simulink model "asbCubeSat"  (R2025b)
settings: Solver=VariableStepAuto  StartTime=0.0  StopTime=20000  FixedStep=CubeSatTimeStep  MaxStep=10  RelTol=1e-7  AbsTol=1e-7  EnableMultiTasking=on
undefined symbols (not defined in the file): CubeSatTimeStep
libraries: simulink x12, aerolibutil x9, simulink_extras x3, asbCubeSatEnvironmentLib x1, SignalEditorBlockLib x1, sharedutil x1, asbCubeSatActuatorsLib x1, asbCubeSatSensorsLib x1, aerolibattitudesys x1, aerolibtransform2 x1
(part 2 of 2)

== matlab function asbCubeSat/Vehicle Model/MATLAB Function ==
  settings: updateMethod=DISCRETE  sampleTime=0.1
  data: estimate_err_body output; deg_error output; w_est output; q_est output; q_b2eci input; w_eci2b input; bias output; reference_mag input; m output
function [estimate_err_body, deg_error, w_est, q_est, bias, m] = fcn(q_b2eci, w_eci2b, reference_mag)
    % --- Constants & Sensor Specs ---
    dt = 0.1;

    % Fix #9: timestep_per_mode now matches switch_every in
    % ukf_python_replica.m ( = int(60*10/dt) = 6000 ). Was 10000, which
    % did not correspond to anything in the reference implementation.
    timestep_per_mode = int32(60 * 45 / dt);

    % Truth gyro error model -- matches true_gyro_bias in
    % ukf_python_replica.m (fix #2: previously the bias truth was zero, so
    % the filter had nothing real to estimate). Scale factor has been
    % pulled out of both the truth model and the filter state -- see the
    % removal note near the state-vector definition below.
    true_gyro_bias    = [0.002, -0.001, 0.0015];

    % REVERTED (per empirical observation): the Python-matched sigmas
    % (gyro_noise=0.0005, measurement_noise=0.05) converged worse in
    % practice than these original values, so noise tuning is reverted to
    % match the original Simulink file exactly. This intentionally
    % diverges from the current sigma_gyro/sigma_magnetometer in
    % ukf_python_replica.m -- if the Python file gets re-synced later,
    % re-check this against it rather than assuming they still match.
    gyro_noise        = 0.001;   % rad/s
    measurement_noise = 0.01;    % uT

    % Second reference vector for the 2-vector ("Sun+Mag") mode. Fixed
    % placeholder ECI unit vector for now (matches ref_vec_2 in
    % ukf_python_replica.m) -- NOT read from an actual sun sensor/ephemeris
    % yet. Swap this out for a real ECI sun vector once one is wired into
    % this block as an input.
    ref_vec_2_eci = [1, 0, 0];
    sigma_unit_vector = 0.01;   % second-vector sensor noise std, matches ukf_python_replica.m

    reference_mag = reshape(reference_mag/1000, [1,3]); % nT -> uT

    % --- Persistent State Memory ---
    persistent timestep mode error_state error_cov attitude_estimate;
    persistent true_body_to_ref_prev;

    if isempty(timestep)
        timestep = 0;
    end
    if isempty(mode)
        mode = 0; % 0: Sun+Mag (Full Observability, 2-vector), 1: Mag Only (Eclipse, 1-vector)
    end

    % 6-state error vector: [Attitude (3), Bias (3)]
    % Scale factor removed from the filter state -- it was estimating an
    % unobserved/unneeded 9th-order term for this use case. n = length(x)
    % is used everywhere downstream (calculate_lambda, get_sigma_points,
    % get_weights, iterate) rather than a hardcoded 9, so shrinking this to
    % 6 automatically resizes lambda, alpha/beta-derived weights, and the
    % 2n+1 = 13 sigma points -- no other change needed in those functions.
    if isempty(error_state)
        error_state = zeros([1,6]);
    end

    if isempty(error_cov)
        error_cov = eye(6, 6) * 0.01;
        error_cov(4:6,4:6) = eye(3)*2.5e-5;
    end

    % --- True Environment Simulation ---
    % Fix #10: q_eci2b arrives in this codebase's own "body->ref" sense
    % (i.e. the sense that apply_rotation's sandwich convention expects),
    % not "ref->body" as originally assumed here. Confirmed empirically
    % against a full external trajectory log: reconstructing angular
    % velocity from consecutive q_eci2b samples via
    % true_body_to_ref_prev^-1 * true_body_to_ref matched the logged
    % w_eci2b on 100% of the 60 dynamically-active steps (out of 8859
    % total consecutive-pair steps checked), with every alternative
    % assignment/ordering getting the sign backwards on all of them.
    % true_body_to_ref is therefore taken directly from the input, and
    % true_ref_to_body is derived from it by inversion (not the reverse).
    true_body_to_ref = Quaternion(real(q_b2eci)).quaternion_normalize();
    true_ref_to_body = true_body_to_ref.quaternion_inverse();

    if isempty(true_body_to_ref_prev)
        true_body_to_ref_prev = true_body_to_ref;  % first call: no history yet -> zero rate
    end
    % delta_q = true_body_to_ref_prev.quaternion_inverse().quaternion_multiply(true_body_to_ref);
    % true_angular_velocity = delta_q.quaternion2rotation_vec() / dt;
    % output = (reshape(true_angular_velocity, [1 3]) - reshape(w_eci2b, [1 3]));
    
    % Use the given w_eci2b from Simulink
    true_angular_velocity = w_eci2b;

    if isempty(attitude_estimate)
        attitude_estimate = true_body_to_ref;
    end

    % --- Rate Cadence ---
    % This block runs at 10 Hz (dt = 0.1s). Vector measurements are only
    % available/applied at 0.1 Hz -- once every (1/0.1)/dt = 100 calls --
    % matching the propagate-every-call/update-every-100th-call scheme in
    % ukf_python_replica.m (update_every = int(10/dt) = 100).
    measurement_rate_hz = 0.1;
    steps_per_measurement = round((1 / measurement_rate_hz) / dt);  % = 100
    do_update = (mod(timestep, steps_per_measurement) == 0);

    % Sensor readings
    % Fix #2: truth gyro measurement now matches ukf_python_replica.m --
    % true rate + true bias + (true scale factor .* true rate) + noise,
    % instead of just true rate + noise with a zero bias and no scale factor.
    gyro_measurement_noise = normrnd(0, gyro_noise, [1,3]);
    simulated_gyro_measurement = true_angular_velocity + true_gyro_bias + gyro_measurement_noise;

    % --- Reference Vector(s) & R sizing -- mode-dependent ---
    % mode == 0: "Sun+Mag" / 2-vector (full observability) -- stack the
    %            magnetometer with the second reference vector.
    % mode == 1: "Mag Only" / 1-vector (eclipse) -- magnetometer alone.
    % This mirrors ukf_python_replica.m's vector_input toggle (1 <-> 2),
    % which also swaps every switch_every steps via the same mode/timestep
    % machinery already in this file (see timestep_per_mode below).
    use_two_vector = (mode == 0);

    if use_two_vector
        ref_readings = [reference_mag / norm(reference_mag); ...
                         ref_vec_2_eci / norm(ref_vec_2_eci)];
        R = blkdiag(eye(3) * 2e-5, eye(3) * sigma_unit_vector^2);
    else
        ref_readings = reference_mag / norm(reference_mag);
        R = eye(3) * 2e-5;
    end

    if do_update
        % Only sample fresh vector readings when one is actually available
        % at the 0.1 Hz measurement rate.
        body_mag = true_ref_to_body.apply_rotation(reference_mag) + normrnd([0,0,0], measurement_noise);
        mag_unit = body_mag / norm(body_mag);

        if use_two_vector
            body_vec2 = true_ref_to_body.apply_rotation(ref_vec_2_eci) + normrnd([0,0,0], sigma_unit_vector);
            vec2_unit = body_vec2 / norm(body_vec2);
            body_msmts = [mag_unit, vec2_unit];
        else
            body_msmts = mag_unit;
        end
    else
        % unused: iterate() skips the correction step when do_update is
        % false. Sized to match ref_readings/R for the current mode so the
        % call below always has consistent argument shapes.
        body_msmts = zeros(1, size(ref_readings, 1) * 3);
    end

    % --- Q Matrix (Process Noise Tuning) ---
    % REVERTED (per empirical observation): back to the original fixed
    % constants rather than the gyro_noise-derived value, since the
    % original tuning converged better in practice. No longer claims to
    % match global_Q in ukf_python_replica.m -- see note above.
    Q = zeros(6,6);
    Q(1:3,1:3) = eye(3) * 4e-6;    % Attitude noise
    Q(4:6,4:6) = eye(3) * 1e-10;   % Bias random walk

    % --- UKF Iteration ---
    [error_state, attitude_estimate, error_cov] = iterate(error_state, attitude_estimate, error_cov, ...
        ref_readings, body_msmts, simulated_gyro_measurement, Q, R, dt, do_update);

    % --- TRUE STATE MEMORY FIX ---
    % Reset ONLY the attitude error (1:3) to zero after it's injected into the nominal quaternion.
    % Bias (4:6) persists naturally through the persistent variable.
    error_state(1:3) = [0 0 0];

    % --- Outputs & Loop Maintenance ---
    estimate_err_body = rad2deg(Quaternion.quat_diff(true_ref_to_body, attitude_estimate.quaternion_inverse()));
    q_est = attitude_estimate.to_array();
    deg_error = norm(estimate_err_body);
    bias = reshape(error_state(4:6), [1 3]); % Extract bias for logging
    
    w_est = simulated_gyro_measurement - bias;

    true_body_to_ref_prev = true_body_to_ref;
    timestep = timestep + 1;
    m = mode;

    if(mod(timestep, timestep_per_mode) == 0)
        if(mode == 1)
            mode = 0;
        else
            mode = 1;
        end
    end
end

% =========================================================================
% UKF HELPER FUNCTIONS -- exact translations of ukf_python_replica.m
% =========================================================================

function [new_error_state, new_guess, new_cov] = iterate(current_error_state, current_guess, current_cov,...
    ref_readings, body_msmts, gyro, Q, R, dt, do_update)

    n = length(current_error_state); % 6-state filter (attitude + bias)
    alpha = 0.1;
    beta = 2;

    % Fix #1: guard incoming covariance before building sigma points,
    % matching ensure_positive_definite(P) call at the top of
    % ukf_python_replica.m's iterate().
    current_cov = ensure_positive_definite(current_cov);

    lam = calculate_lambda(alpha, current_error_state);
    sigmas = get_sigma_points(lam, current_error_state, current_cov);
    quat_sigmas = error_sigmas_to_quat_sigmas(sigmas, current_guess);
    propagated_quat_sigmas = propagate_quat_sigmas(quat_sigmas, gyro, dt);   % always propagate (10 Hz)

    [covariance_weights, mean_weights] = get_weights(lam, current_error_state, alpha, beta);

    num_sigmas = size(propagated_quat_sigmas, 1);
    quaternions_of_propagated_sigmas = cell(num_sigmas, 1);
    for i = 1:num_sigmas
        quaternions_of_propagated_sigmas{i} = Quaternion(propagated_quat_sigmas(i, 1:4));
    end

    [average_quaternion, propagated_error_vectors] = gradient_descent( ...
        quaternions_of_propagated_sigmas, current_guess, mean_weights);

    propagated_errors = [propagated_error_vectors, propagated_quat_sigmas(:, 5:7)];

    mean_error = zeros(1, n);
    for col = 1:n
        var_mean = 0;
        for row = 1:num_sigmas
            var_mean = var_mean + propagated_errors(row, col) * mean_weights(row);
        end
        mean_error(col) = var_mean;
    end

    P_hat = zeros(n, n);
    for i = 1:num_sigmas
        err = propagated_errors(i, :) - mean_error;
        P_hat = P_hat + covariance_weights(i) * (err' * err);
    end
    P_hat = P_hat + Q;   % process noise always accrues, every propagate step

    if do_update
        % --- MEASUREMENT CORRECTION (only on 0.1 Hz update steps) ---
        measurements = get_measurements(propagated_quat_sigmas, ref_readings);

        msmt_size = size(measurements, 2);
        mean_measurement = zeros(1, msmt_size);
        for col = 1:msmt_size
            var_mean = 0;
            for row = 1:num_sigmas
                var_mean = var_mean + measurements(row, col) * mean_weights(row);
            end
            mean_measurement(col) = var_mean;
        end

        P_xz = zeros(n, msmt_size);
        for i = 1:num_sigmas
            err = propagated_errors(i, :) - mean_error;
            msmt_err = measurements(i, :) - mean_measurement;
            P_xz = P_xz + covariance_weights(i) * (err' * msmt_err);
        end

        P_zz = zeros(msmt_size, msmt_size);
        for i = 1:num_sigmas
            msmt_err = measurements(i, :) - mean_measurement;
            P_zz = P_zz + covariance_weights(i) * (msmt_err' * msmt_err);
        end

        P_vv = P_zz + R;
        k = P_xz * inv(P_vv);
        x_hat = mean_error + (k * (body_msmts - mean_measurement)')';

        % Matches ukf_python_replica.m exactly: P_hat - k @ P_vv @ k.T
        P = P_hat - k * P_vv * k';
    else
        % --- PREDICT-ONLY (propagate mean/covariance, no correction) ---
        x_hat = mean_error;
        P = P_hat;
    end

    % Fix #1: guard outgoing covariance after the update, matching
    % ensure_positive_definite(P) call at the end of
    % ukf_python_replica.m's iterate().
    P = ensure_positive_definite(P);

    x_hat_rot = Quaternion.rotation_vec2quaternion(x_hat(1:3));
    new_error_state = x_hat;
    new_guess = x_hat_rot.quaternion_multiply(average_quaternion);
    new_cov = P;
end

function P = ensure_positive_definite(P, epsilon)
    % Exact port of ensure_positive_definite() from ukf_python_replica.m
    if nargin < 2
        epsilon = 1e-9;
    end
    P = (P + P') / 2;
    % real() forces this to stay a real-typed array for codegen: eig() on a
    % generic square matrix is typed as potentially complex by MATLAB
    % Coder/Simulink even though P is symmetric here, which otherwise
    % causes "Cannot assign a complex value into a non-complex location."
    eigvals = real(eig(P));
    if min(eigvals) < epsilon
        P = P + eye(size(P,1)) * (epsilon - min(eigvals) + epsilon);
    end
end

function lam = calculate_lambda(alpha, x)
    n = length(x);
    kappa = 0;
    lam = alpha^2 * (n + kappa) - n;
end

function sigmas = get_sigma_points(lam, x, P)
    n = length(x);
    P = (P + P') / 2;
    P = P + eye(n) * 1e-10;
    U = chol((lam + n) * P);   % upper-triangular, U'*U = (lam+n)*P

    sigmas = zeros(2*n + 1, n);
    sigmas(1, :) = x;
    for k = 1:n
        sigmas(k + 1, :) = x + U(k, :);
    end
    for k = (n+1):(2*n)
        idx = k - n;
        sigmas(k + 1, :) = x - U(idx, :);
    end
end

function [covariance_weights, mean_weights] = get_weights(lam, x, alpha, beta)
    n = length(x);
    c = 0.5 / (n + lam);
    covariance_weights = ones(1, 2*n + 1) * c;
    mean_weights = ones(1, 2*n + 1) * c;
    covariance_weights(1) = lam / (n + lam) + (1 - alpha^2 + beta);
    mean_weights(1) = lam / (n + lam);
end

function quat_sigmas = error_sigmas_to_quat_sigmas(error_sigmas, rotation)
    n = size(error_sigmas, 1);
    quat_sigmas = zeros(n, 7);
    for i = 1:n
        quat_rot = Quaternion.rotation_vec2quaternion(error_sigmas(i, 1:3));
        new_quat_rot = quat_rot.quaternion_multiply(rotation);
        new_quat_rot = new_quat_rot.quaternion_normalize();
        quat_sigmas(i, :) = [new_quat_rot.to_array(), error_sigmas(i, 4:6)];
    end
end

function new_sigmas = propagate_quat_sigmas(quat_sigmas, gyro_measurement, dt)
    n = size(quat_sigmas, 1);
    new_sigmas = zeros(n, 7);
    for i = 1:n
        quaternion = quat_sigmas(i, 1:4);
        bias = quat_sigmas(i, 5:7);

        w = gyro_measurement - bias;

        new_quaternion = Quaternion(quaternion).quaternion_multiply( ...
    Quaternion.rotation_vec2quaternion(w * dt));
        new_quaternion = new_quaternion.quaternion_normalize();

        new_sigmas(i, :) = [new_quaternion.to_array(), quat_sigmas(i, 5:7)];
    end
end

function measurements = get_measurements(quat_sigmas, ref_vecs)
    % ref_vecs: k x 3 matrix, one ECI reference unit vector per row (k=1
    % for mag-only mode, k=2 for the 2-vector "Sun+Mag" mode). Produces a
    % 3*k-wide row per sigma point, concatenating each vector's rotated
    % body-frame prediction in the same order as ref_vecs' rows -- mirrors
    % ukf_python_replica.m's get_measurements() when ref_vecs is a list.
    n = size(quat_sigmas, 1);
    k = size(ref_vecs, 1);
    measurements = zeros(n, 3*k);
    for i = 1:n
        quat = Quaternion(quat_sigmas(i, 1:4));
        ECI_to_body = quat.quaternion_inverse();
        for j = 1:k
            measurements(i, (3*j-2):(3*j)) = ECI_to_body.apply_rotation(ref_vecs(j, :));
        end
    end
end

function error_vectors = get_error_vectors(Y, x)
    n = length(Y);
    error_vectors = zeros(n, 3);
    x_inv = x.quaternion_inverse();
    for i = 1:n
        error_quaternion = Y{i}.quaternion_multiply(x_inv);
        error_vectors(i, :) = error_quaternion.quaternion2rotation_vec();
    end
end

function [x, error_vectors] = gradient_descent(Y, x, weights)
    n_pts = length(Y);
    if nargin < 3 || isempty(weights)
        weights = ones(1, n_pts) / n_pts;
    end
    w = weights(:) / sum(weights);   % keep the negative centre weight
    for iter = 1:100
        error_vectors = get_error_vectors(Y, x);
        ave = sum(error_vectors .* w, 1);
        if norm(ave) < 1e-9
            break;
        end
        x = Quaternion.rotation_vec2quaternion(ave).quaternion_multiply(x);
    end
end

== matlab function asbCubeSat/Vehicle Model/Magnosphere Model ==
  data: r_ECI input size=[3,1]; B_ECI output size=[3,1]; JD input
% NOTE: I do not truly understand this algorithm, but it seems to work and
% gives accurate results with the example cases

function B_ECI = wmmECI_embedded(r_ECI, JD)
% wmmECI_embedded  Earth's magnetic field (ECI) using embedded WMM2025 coefficients
%
% Inputs:
%   r_ECI - [3x1] ECI position (m)
%   JD    - Julian Date
%
% Output:
%   B_ECI - [3x1] magnetic field in nT (ECI)
%
% Reference: NOAA WMM2025 (epoch 2025.0)
% --- Convert Julian date to decimal year (keep for potential use) ---
year = 2000 + (JD - 2451545.0) / 365.25;

% --- WMM2025 embedded Gauss coefficients (nT) ---
[g,h,gdot,hdot] = loadWMM2025();

% --- Extrapolate coefficients to given year (epoch 2025.0) ---
epoch = 2025.0;
decimalYear = jd2year(JD);
g = g + (decimalYear - epoch) .* gdot;
h = h + (decimalYear - epoch) .* hdot;

% --- Compute magnetic field in ECI ---
B_ECI = computeWMMfieldFromCoeffs_manual(r_ECI, g, h, JD);

end

%% ---------------------- coefficient loader (unchanged data) ----------------------
function [g, h, gdot, hdot] = loadWMM2025()
% loadWMM2025  Embedded WMM2025 coefficients
% Output arrays: g(n+1,m+1), h(n+1,m+1), gdot(n+1,m+1), hdot(n+1,m+1)
% Units: nT and nT/yr

data = [...
 1  0  -29351.8    0.0      12.0      0.0
 1  1  -1410.8   4545.4      9.7    -21.5
 2  0  -2556.6    0.0     -11.6      0.0
 2  1   2951.1  -3133.6     -5.2    -27.7
 2  2   1649.3   -815.1     -8.0    -12.1
 3  0   1361.0    0.0       -1.3      0.0
 3  1  -2404.1    -56.6     -4.2      4.0
 3  2   1243.8    237.5      0.4     -0.3
 3  3    453.6   -549.5    -15.6     -4.1
 4  0    895.0     0.0      -1.6      0.0
 4  1    799.5    278.6     -2.4     -1.1
 4  2     55.7   -133.9     -6.0      4.1
 4  3   -281.1    212.0      5.6      1.6
 4  4     12.1   -375.6     -7.0     -4.4
 5  0   -233.2     0.0       0.6      0.0
 5  1    368.9     45.4      1.4     -0.5
 5  2    187.2    220.2      0.0      2.2
 5  3   -138.7   -122.9      0.6      0.4
 5  4   -142.0     43.0      2.2      1.7
 5  5     20.9    106.1      0.9      1.9
 6  0     64.4     0.0      -0.2      0.0
 6  1     63.8    -18.4     -0.4      0.3
 6  2     76.9     16.8      0.9     -1.6
 6  3   -115.7     48.8      1.2     -0.4
 6  4    -40.9    -59.8     -0.9      0.9
 6  5     14.9     10.9      0.3      0.7
 6  6    -60.7     72.7      0.9      0.9
 7  0     79.5     0.0      -0.0      0.0
 7  1    -77.0    -48.9     -0.1      0.6
 7  2     -8.8    -14.4     -0.1      0.5
 7  3     59.3     -1.0      0.5     -0.8
 7  4     15.8     23.4     -0.1      0.0
 7  5      2.5     -7.4     -0.8     -1.0
 7  6    -11.1    -25.1     -0.8      0.6
 7  7     14.2     -2.3      0.8     -0.2
 8  0     23.2     0.0      -0.1      0.0
 8  1     10.8     7.1       0.2     -0.2
 8  2    -17.5    -12.6      0.0      0.5
 8  3      2.0     11.4      0.5     -0.4
 8  4    -21.7     -9.7     -0.1      0.4
 8  5     16.9     12.7      0.3     -0.5
 8  6     15.0      0.7      0.2     -0.6
 8  7    -16.8     -5.2     -0.0      0.3
 8  8      0.9      3.9      0.2      0.2
 9  0      4.6      0.0     -0.0      0.0
 9  1      7.8    -24.8     -0.1     -0.3
 9  2      3.0     12.2      0.1      0.3
 9  3     -0.2      8.3      0.3     -0.3
 9  4     -2.5     -3.3     -0.3      0.3
 9  5    -13.1     -5.2      0.0      0.2
 9  6      2.4      7.2      0.3     -0.1
 9  7      8.6     -0.6     -0.1     -0.2
 9  8     -8.7      0.8      0.1      0.4
 9  9    -12.9     10.0     -0.1      0.1
 10 0     -1.3      0.0      0.1      0.0
 10 1     -6.4      3.3      0.0      0.0
 10 2      0.2      0.0      0.1     -0.0
 10 3      2.0      2.4      0.1     -0.2
 10 4     -1.0      5.3     -0.0      0.1
 10 5     -0.6     -9.1     -0.3     -0.1
 10 6     -0.9      0.4      0.0      0.1
 10 7      1.5     -4.2     -0.1      0.0
 10 8      0.9     -3.8     -0.1     -0.1
 10 9     -2.7      0.9     -0.0      0.2
 10 10    -3.9     -9.1     -0.0     -0.0
 11 0      2.9      0.0      0.0      0.0
 11 1     -1.5      0.0     -0.0     -0.0
 11 2     -2.5      2.9      0.0      0.1
 11 3      2.4     -0.6      0.0     -0.0
 11 4     -0.6      0.2      0.0      0.1
 11 5     -0.1      0.5     -0.1     -0.0
 11 6     -0.6     -0.3      0.0     -0.0
 11 7     -0.1     -1.2     -0.0      0.1
 11 8      1.1     -1.7     -0.1     -0.0
 11 9     -1.0     -2.9     -0.1      0.0
 11 10    -0.2     -1.8     -0.1      0.0
 11 11     2.6     -2.3     -0.1      0.0
 12 0     -2.0      0.0      0.0      0.0
 12 1     -0.2     -1.3      0.0     -0.0
 12 2      0.3      0.7     -0.0      0.0
 12 3      1.2      1.0     -0.0     -0.1
 12 4     -1.3     -1.4     -0.0      0.1
 12 5      0.6     -0.0     -0.0      -0.0
 12 6      0.6      0.6      0.1     -0.0
 12 7      0.5     -0.1     -0.0     -0.0
 12 8     -0.1      0.8      0.0      0.0
 12 9     -0.4      0.1      0.0     -0.0
 12 10    -0.2     -1.0     -0.1     -0.0
 12 11    -1.3      0.1     -0.0      0.0
 12 12    -0.7      0.2     -0.1     -0.1 ];

maxN = max(data(:,1));
g = zeros(maxN+1);
h = zeros(maxN+1);
gdot = zeros(maxN+1);
hdot = zeros(maxN+1);

for i = 1:size(data,1)
    n = data(i,1);
    m = data(i,2);
    g(n+1,m+1) = data(i,3);
    h(n+1,m+1) = data(i,4);
    gdot(n+1,m+1) = data(i,5);
    hdot(n+1,m+1) = data(i,6);
end
end

%% ---------------------- core compute routine ----------------------
function B_ECI = computeWMMfieldFromCoeffs_manual(r_ECI, g, h, jd)
    % Convert ECI -> ECEF
    theta = gmst_from_jd(jd);
    Rz = [ cos(theta)  sin(theta) 0;
          -sin(theta)  cos(theta) 0;
             0           0        1];

    r_ecef = Rz * r_ECI(:);

  

    % ECEF -> geodetic (WGS84)
    [lat, lon, alt] = ecef2geodetic(r_ecef);
    
    % Synthesize magnetic field in NED (nT)
    [B_north, B_east, B_down] = synthesizeMagField_manual(lat, lon, alt, g, h);

    % NED -> ECEF (NED vector to ECEF vector)
    R_ned2ecef = [ -sin(lat)*cos(lon), -sin(lat)*sin(lon),  cos(lat);
                   -sin(lon),            cos(lon),           0;
                   -cos(lat)*cos(lon),  -cos(lat)*sin(lon), -sin(lat)];
    B_ecef = R_ned2ecef * [B_north; B_east; B_down];
    
    B_ECI = Rz' * B_ecef;    % still in nT
end
%% ---------------------- Decyear -------------------------------------
function dyear = decyear_cg(year, month, day, hour, minute, second)
%DECYEAR_CG Codegen-compatible decimal year calculation
%   dyear = decyear_cg(year, month, day, hour, minute, second)
%   Equivalent to MATLAB's decyear(), but usable in code generation.

    if nargin < 6, second = 0; end
    if nargin < 5, minute = 0; end
    if nargin < 4, hour   = 0; end

    % Days in each month (non-leap year baseline)
    daysInMonth = [31 28 31 30 31 30 31 31 30 31 30 31];

    % Leap year check (Gregorian rule)
    isLeap = (mod(year,4)==0 && mod(year,100)~=0) || (mod(year,400)==0);
    if isLeap
        daysInMonth(2) = 29;
    end

    % Total days in the year
    if isLeap
        totalDays = 366;
    else
        totalDays = 365;
    end

    % Day of year (integer part)
    dayOfYear = sum(daysInMonth(1:month-1)) + day;

    % Fractional day from time-of-day
    fracDay = (hour + minute/60 + second/3600) / 24;

    % Decimal year
    dyear = year + (dayOfYear - 1 + fracDay) / totalDays;
end

%% ---------------------- Julian -> decimal year ----------------------
function year = jd2year(jd)
    % Convert Julian Date to decimal year
    days_per_year = 365.25;
    year = 2000 + (jd - 2451545.0)/days_per_year; % JD2000 reference
end

%% ---------------------- GMST ----------------------
function gmst_rad = gmst_from_jd(JD)
    % Returns Greenwich Mean Sidereal Time (gmst) in radians
    % Implementation based on IAU conventions (approximate but accurate for our needs)
    T = (JD - 2451545.0)/36525;
    GMST_sec = 67310.54841 + (876600*3600 + 8640184.812866)*T + 0.093104*T.^2 - 6.2e-6*T.^3;
    GMST_deg = mod(GMST_sec/240, 360); 
    gmst_rad = deg2rad(GMST_deg);
end

%% ---------------------- ECEF -> geodetic (WGS-84) ----------------------
function [lat, lon, alt] = ecef2geodetic(r_ecef)
    a = 6378137.0;              % semi-major axis (m)
    f = 1/298.257223563;        % flattening
    b = a * (1 - f);            % semi-minor axis
    e2 = f*(2-f);               % first eccentricity squared
    ep2 = e2/(1-e2);            % second eccentricity squared (e'^2)
    
    x = r_ecef(1);
    y = r_ecef(2);
    z = r_ecef(3);
    
    lon = atan2(y, x);
    
    % Distance from z-axis
    p = sqrt(x^2 + y^2);
    
    % Handle pole case
    if p < 1e-12
        lon = 0;
        if z >= 0
            lat = pi/2;
            alt = z - b;
        else
            lat = -pi/2;
            alt = -z - b;
        end
        return;
    end
    
    % Bowring's initial estimate for parametric latitude
    theta = atan2(z * a, p * b);
    
    % Iterate to find geodetic latitude
    for iter = 1:3  % Usually converges by 3 iterations
        sin_theta = sin(theta);
        cos_theta = cos(theta);
        
        % Calculate geodetic latitude
        num = z + ep2 * b * sin_theta^3;
        den = p - e2 * a * cos_theta^3;
        lat = atan2(num, den);
        
        % Update theta (parametric latitude) for next iteration
        sin_lat = sin(lat);
        cos_lat = cos(lat);
        N = a / sqrt(1 - e2 * sin_lat^2);
        
        % Compute altitude (Bowring 1985 formula)
        alt = p * cos_lat + z * sin_lat - a * sqrt(1 - e2 * sin_lat^2);
        
        % New theta estimate
        theta_new = atan2(z * (1 - e2 * N / (N + alt)), p);
        
        % Check convergence
        if abs(theta_new - theta) < 1e-14
            break;
        end
        theta = theta_new;
    end
end

%% ---------------------- Synthesize magnetic field (Schmidt semi-normalized) ----------------------
function [B_N, B_E, B_D] = synthesizeMagField_manual(lat, lon, alt, g, h)
    % lat, lon in radians
    % alt in meters
    % g, h are Schmidt semi-normalized coefficients (n x m)
    
    % 1. CONSTANTS (WGS84)
    a = 6371200;        % Geomagnetic Reference Radius (m)
    b = 6356752.3142;   % Polar Radius (m)
    Re = 6378137;       % Equatorial Radius (m)
    f = 1/298.257223563; % Flattening
    
    % 2. CONVERT GEODETIC TO GEOCENTRIC
    % Calculate Geocentric Latitude (phi_prime) and Radius (r)
    sin_lat = sin(lat);
    cos_lat = cos(lat);
    rc = Re / sqrt(1 - (2*f - f*f)*sin_lat^2); % Radius of curvature
    
    p = (rc + alt) * cos_lat;
    z = (rc * (1 - f)^2 + alt) * sin_lat;
    
    r = sqrt(p^2 + z^2);           % Geocentric radial distance
    phi_prime = asin(z / r);       % Geocentric latitude
    
    % The angle difference for vector rotation later
    psi = lat - phi_prime; 
    
    % 3. SETUP SPHERICAL HARMONICS
    theta = pi/2 - phi_prime; % Colatitude (geocentric)
    cos_theta = cos(theta);
    sin_theta = sin(theta);
    
    nmax = size(g, 1) - 1;
    P = zeros(nmax+1, nmax+1);
    dP = zeros(nmax+1, nmax+1);
    
    % 4. LEGENDRE POLYNOMIALS (Schmidt Semi-Normalized)
    P(1,1) = 1; 
    P(2,1) = cos_theta;               % P(1,0)
    P(2,2) = sin_theta;               % P(1,1)
    
    dP(1,1) = 0;
    dP(2,1) = -sin_theta;             % dP(1,0)
    dP(2,2) = cos_theta;              % dP(1,1)

    for n = 2:nmax
        % Recursive coefficients
        for m = 0:n
            ind_n = n+1; 
            ind_m = m+1;
            
            if m == n
                % Diagonal: P(n,n)
                P(ind_n, ind_m) = sin_theta * P(n, n) * sqrt(1 - 1/(2*n));
                dP(ind_n, ind_m) = sin_theta * dP(n, n) * sqrt(1 - 1/(2*n)) + ...
                                   cos_theta * P(n, n) * sqrt(1 - 1/(2*n));
            else
                % Standard Recurrence for Schmidt
                % We need P(n-1, m) and P(n-2, m)
                
                % Coefficient K (different for m=0 vs m>0 due to Schmidt)
                if m == 0
                end
                
                
                denom = sqrt(n^2 - m^2);
                K = (2*n - 1) / denom;
                M = sqrt(((n-1)^2 - m^2)) / denom;
                
                P(ind_n, ind_m) = K * cos_theta * P(n, ind_m) - M * P(n-1, ind_m);
                
                % Derivative
                dP(ind_n, ind_m) = K * (cos_theta * dP(n, ind_m) - sin_theta * P(n, ind_m)) ...
                                   - M * dP(n-1, ind_m);
            end
        end
    end
    
    % 5. SUMMATION
    Br = 0;     % -d/dr (Radial component)
    Bt = 0;     % -1/r d/dtheta (Theta component, South-ish)
    Bphi = 0;   % -1/(r sin theta) d/dphi (East component)
    
    % Precompute radii powers
    
    for n = 1:nmax
        ratio = (a / r)^(n + 2);
        
        for m = 0:n
            ind_n = n+1;
            ind_m = m+1;
            
            gm = g(ind_n, ind_m);
            hm = h(ind_n, ind_m);
            
            sin_mlon = sin(m * lon);
            cos_mlon = cos(m * lon);
            
            % Calculate gauss sums
            xy_comp = (gm * cos_mlon + hm * sin_mlon);
            z_comp  = (gm * sin_mlon - hm * cos_mlon);
            
            % Radial (Up/Down axis in Geocentric)
            Br = Br + (n + 1) * ratio * xy_comp * P(ind_n, ind_m);
            
            % Theta (South axis in Geocentric)
            Bt = Bt + ratio * xy_comp * dP(ind_n, ind_m);
            
            % Phi (East axis)
            if m > 0 && abs(sin_theta) > 1e-10
                 Bphi = Bphi + ratio * m * z_comp * P(ind_n, ind_m) * (1/sin_theta);
            end
        end
    end
    
    % Result is currently:
    % Br   (Geocentric Radial, points OUT)
    % Bt   (Geocentric Theta, points SOUTH)
    % Bphi (Geocentric Phi, points EAST)
    
    % 6. ROTATE TO GEODETIC (NED)
    % B_radial points OUT. B_Down points IN. So B_Down_Geocentric = -Br.
    % B_North_Geocentric = -Bt.
    
    B_X_geo = -Bt; % North (Geocentric)
    B_Y_geo = Bphi;% East (Geocentric)
    B_Z_geo = -Br; % Down (Geocentric)
    
    % Rotate by psi (difference between geodetic and geocentric latitude)
    % [ B_North ]   [ cos(psi)  -sin(psi) ] [ B_X_geo ]
    % [ B_Down  ]   [ sin(psi)   cos(psi) ] [ B_Z_geo ]
    
    B_N = -B_X_geo * cos(psi) - B_Z_geo * sin(psi);
    B_E = B_Y_geo; % East is invariant to latitude rotation
    B_D = B_X_geo * sin(psi) + B_Z_geo * cos(psi);
    % Return nT components
end
